simulink model "C_sim"  (R2024b)
settings: Solver=VariableStepAuto  StartTime=0.0  StopTime=ncs.simTime  FixedStep=Td  RelTol=1e-3
InitFcn:
  | set_param(gcs, 'SimulationCommand', 'update')
values from neighbouring files (symbols this model uses):
  ncs = NcsStructure(ncsPlant, 'simTime', simulationTime, 'controlParams', controlParams)    [main.m]
undefined symbols (not defined in the file or in its folder): sfunchk
libraries: cstblocks x1, truetime x1
settings Model: Creator=jakob_ludwiger  LastModifiedBy=proph37
settings SolverCC: AlgebraicLoopSolver=TrustRegion
settings DataIOCC: ReturnWorkspaceOutputs=off
settings DebuggingCC: UnconnectedInputMsg=warning  UnconnectedOutputMsg=warning  UnconnectedLineMsg=warning  ArithmeticOperatorsInVariantConditions=warning
settings ModelReferenceCC: EnableRefExpFcnMdlSchedulingChecks=on
settings SFSimCC: SimUseLocalCustomCode=off  CustomCodeUndefinedFunction=UseInterfaceOnly
settings RTWCC: RTWUseLocalCustomCode=off  GPUComputeCapability=3.5  DLArmComputeVersion=19.05
settings CodeAppCC: StateflowObjectComments=on

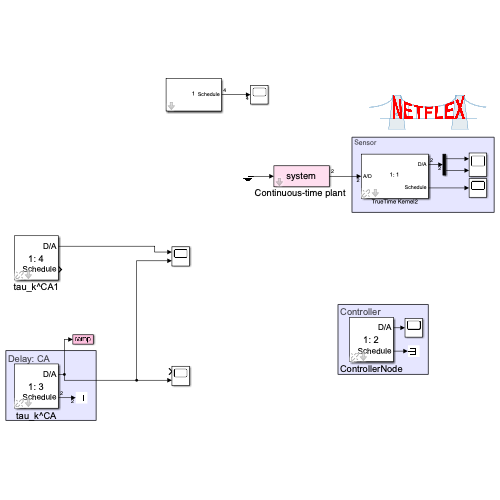
[thumbnail: Simulink's stored preview of the top-level diagram]
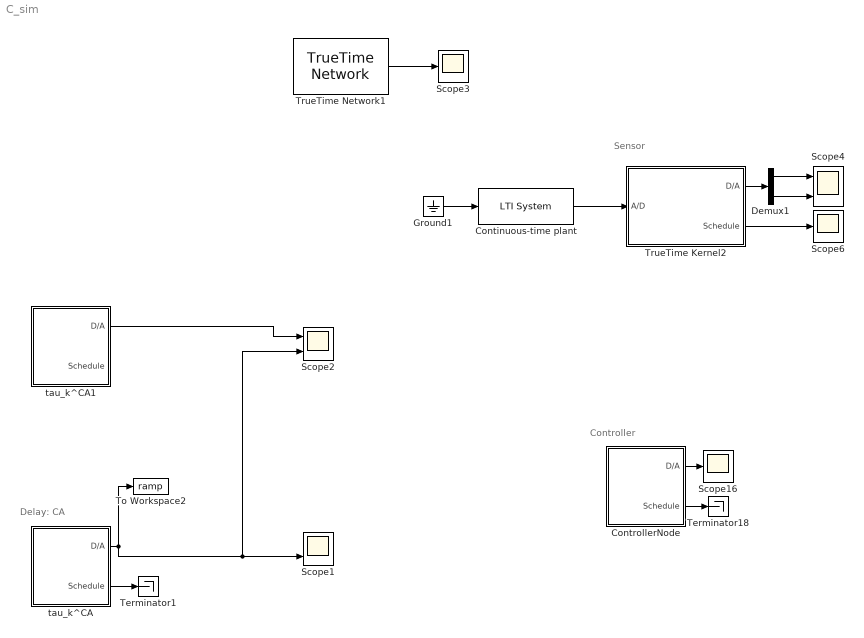
== system C_sim ==
  note: Controller
  note: Sensor
  note: Delay: CA
  "Continuous-time plant " : cstblocks/LTI System  sys=system  IC=initialState  PadeOrder=0
  ControllerNode : Subsystem  AncestorBlock=truetime/TrueTime Kernel  InitFcn=sfunchk(get_param(gcb,'sfun'));  mask{nodeObj=ncs.controllerNode, sfun=initFctWrapper, ntriggers=0, trigtype=falling, clockoffsetdrift=[0 0], schedoutput=on, battery=off, poweroutput=off, label=1: 2}
      mask prompts: nodeObj "Node Object"; sfun "Name of init function (MEX or MATLAB):"; ntriggers "Number of external triggers:"; trigtype "Trigger type:"; clockoffsetdrift "Local clock offset and drift:"; schedoutput "Show Schedule output port"; battery "Show Energy supply input port"; poweroutput "Show Power consumption output port"
      mask init:
      | set_param(gcb,'sfun', nodeObj.initFunctionWrapper)
      | %set_param(gcb,'args', [3 2])
      | args = nodeObj;
      | ninputsoutputs = [nodeObj.Nin nodeObj.Nout];
      | nwnodenbr = nodeObj.nodenumber;
      | ttkernel_callback(gcb,{sfun,args,ninputsoutputs,ntriggers,trigtype,nwnodenbr,clockoffsetdrift,schedoutput,battery,poweroutput})
      settings: ErrorFcn=ttkernel_error
      mask TypeOptions trigtype: rising | falling | either
      mask Display: disp(get_param(gcb,'label'))
  Demux1 : Demux  Outputs=2
  Ground1 : Ground
  Scope1 : Scope  NumInputPorts=2
  Scope16 : Scope
  Scope2 : Scope  NumInputPorts=2
  Scope3 : Scope
  Scope4 : Scope  NumInputPorts=2
  Scope6 : Scope
  Terminator1 : Terminator
  Terminator18 : Terminator
  To Workspace2 : ToWorkspace  VariableName=ramp  SaveFormat=Timeseries  SampleTime=1e-5
  TrueTime Kernel2 : Subsystem  AncestorBlock=truetime/TrueTime Kernel  InitFcn=sfunchk(get_param(gcb,'sfun'));  mask{nodeObj=ncs.sensorNode, sfun=initFctWrapper, ntriggers=0, trigtype=falling, clockoffsetdrift=[0 0], schedoutput=on, battery=off, poweroutput=off, label=1: 1}
      mask prompts: nodeObj "Node Object"; sfun "Name of init function (MEX or MATLAB):"; ntriggers "Number of external triggers:"; trigtype "Trigger type:"; clockoffsetdrift "Local clock offset and drift:"; schedoutput "Show Schedule output port"; battery "Show Energy supply input port"; poweroutput "Show Power consumption output port"
      mask init: same as C_sim/ControllerNode
      settings: ErrorFcn=ttkernel_error
      mask TypeOptions trigtype: rising | falling | either
      mask Display: disp(get_param(gcb,'label'))
  TrueTime Network1 : truetime/TrueTime Network  nwtype=CSMA/CD (Ethernet)  nwnbr=1  nnodes=ncs.getMaxNodeNumber  rate=1e8  minsize=200  lossprob=0  seed=0  bandwidths=[0.5 0.5]  slotsize=512  schedule=[1 1 2]  memsize=80000  buftype=Common buffer  overflow=Retransmit  dynSchedule=0  miniSlotSize=0  NIT=0  QSortMode=FIFO  sync=0  irtSchedule=0  nrtLength=0  nodeGraph=0  scheduleoutput=on
  tau_k^CA : Subsystem  AncestorBlock=truetime/TrueTime Kernel  InitFcn=sfunchk(get_param(gcb,'sfun'));  mask{nodeObj=ncs.tauCaNode, sfun=initFctWrapper, ntriggers=0, trigtype=falling, clockoffsetdrift=[0 0], schedoutput=on, battery=off, poweroutput=off, label=1: 3}
      mask prompts: nodeObj "Node Object"; sfun "Name of init function (MEX or MATLAB):"; ntriggers "Number of external triggers:"; trigtype "Trigger type:"; clockoffsetdrift "Local clock offset and drift:"; schedoutput "Show Schedule output port"; battery "Show Energy supply input port"; poweroutput "Show Power consumption output port"
      mask init: same as C_sim/ControllerNode
      settings: ErrorFcn=ttkernel_error
      mask TypeOptions trigtype: rising | falling | either
      mask Display: disp(get_param(gcb,'label'))
  tau_k^CA1 : Subsystem  AncestorBlock=truetime/TrueTime Kernel  InitFcn=sfunchk(get_param(gcb,'sfun'));  mask{nodeObj=ncs.test1, sfun=initFctWrapper, ntriggers=0, trigtype=falling, clockoffsetdrift=[0 0], schedoutput=on, battery=off, poweroutput=off, label=1: 4}
      mask prompts: nodeObj "Node Object"; sfun "Name of init function (MEX or MATLAB):"; ntriggers "Number of external triggers:"; trigtype "Trigger type:"; clockoffsetdrift "Local clock offset and drift:"; schedoutput "Show Schedule output port"; battery "Show Energy supply input port"; poweroutput "Show Power consumption output port"
      mask init: same as C_sim/ControllerNode
      settings: ErrorFcn=ttkernel_error
      mask TypeOptions trigtype: rising | falling | either
      mask Display: disp(get_param(gcb,'label'))
  wires:
  TrueTime Network1/1 -> Scope3/1
  TrueTime Kernel2/2(Schedule) -> Scope6/1
  Demux1/2 -> Scope4/2
  Ground1/1 -> "Continuous-time plant "/1
  ControllerNode/1(D/A) -> Scope16/1
  "Continuous-time plant "/1 -> TrueTime Kernel2/1(A/D)
  ControllerNode/2(Schedule) -> Terminator18/1
  TrueTime Kernel2/1(D/A) -> Demux1/1
  Demux1/1 -> Scope4/1
  tau_k^CA/1(D/A) -> To Workspace2/1, Scope2/2, Scope1/2
  tau_k^CA/2(Schedule) -> Terminator1/1
  tau_k^CA1/1(D/A) -> Scope2/1

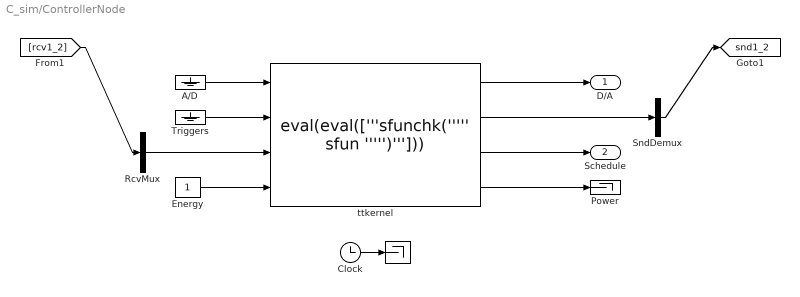
== system C_sim/ControllerNode ==
  " " : Terminator
  A/D : Ground
  Clock : Clock
  Energy : Constant
  Power : Terminator
  RcvMux : Mux  Inputs=1
  SndDemux : Demux  Outputs=1
      settings: DisplayOption=none
  Triggers : Ground
  ttkernel : S-Function  FunctionName=eval(eval(['''sfunchk(''''' sfun ''''')''']))  Parameters=sfun, args, ninputsoutputs, ntriggers, trigtype, nwnodenbr, clockoffsetdrift  SFunctionDeploymentMode=off  EnableBusSupport=off
  D/A : Outport
  Schedule : Outport  Port=2
  tag scope: snd1_2=global
  wires:
  Clock/1 -> " "/1
  RcvMux/1 -> ttkernel/3
  Triggers/1 -> ttkernel/2
  ttkernel/3 -> Schedule/1
  ttkernel/1 -> D/A/1
  ttkernel/2 -> SndDemux/1
  A/D/1 -> ttkernel/1
  Energy/1 -> ttkernel/4
  ttkernel/4 -> Power/1
  [rcv1_2] -> RcvMux/1
  SndDemux/1 -> [snd1_2]

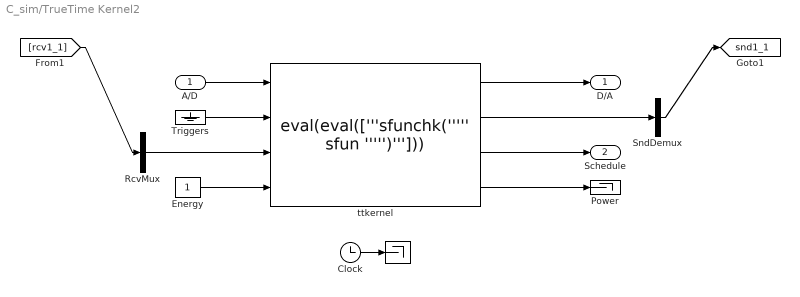
== system C_sim/TrueTime Kernel2 ==
  A/D : Inport
  " " : Terminator
  Clock : Clock
  Energy : Constant
  Power : Terminator
  RcvMux : Mux  Inputs=1
  SndDemux : Demux  Outputs=1
      settings: DisplayOption=none
  Triggers : Ground
  ttkernel : S-Function  FunctionName=eval(eval(['''sfunchk(''''' sfun ''''')''']))  Parameters=sfun, args, ninputsoutputs, ntriggers, trigtype, nwnodenbr, clockoffsetdrift  SFunctionDeploymentMode=off  EnableBusSupport=off
  D/A : Outport
  Schedule : Outport  Port=2
  tag scope: snd1_1=global
  wires:
  ttkernel/4 -> Power/1
  Energy/1 -> ttkernel/4
  A/D/1 -> ttkernel/1
  ttkernel/2 -> SndDemux/1
  ttkernel/1 -> D/A/1
  ttkernel/3 -> Schedule/1
  Triggers/1 -> ttkernel/2
  RcvMux/1 -> ttkernel/3
  Clock/1 -> " "/1
  [rcv1_1] -> RcvMux/1
  SndDemux/1 -> [snd1_1]

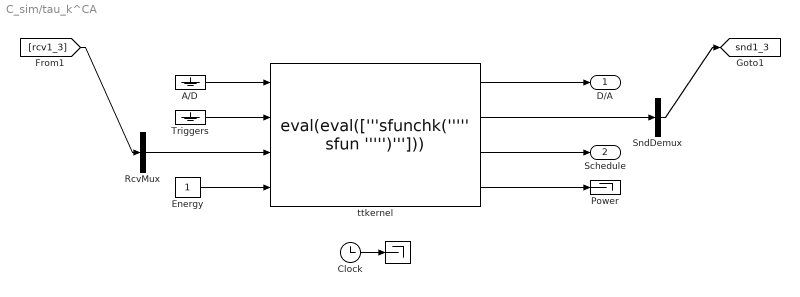
== system C_sim/tau_k^CA ==
  " " : Terminator
  A/D : Ground
  Clock : Clock
  Energy : Constant
  Power : Terminator
  RcvMux : Mux  Inputs=1
  SndDemux : Demux  Outputs=1
      settings: DisplayOption=none
  Triggers : Ground
  ttkernel : S-Function  FunctionName=eval(eval(['''sfunchk(''''' sfun ''''')''']))  Parameters=sfun, args, ninputsoutputs, ntriggers, trigtype, nwnodenbr, clockoffsetdrift  SFunctionDeploymentMode=off  EnableBusSupport=off
  D/A : Outport
  Schedule : Outport  Port=2
  tag scope: snd1_3=global
  wires:
  ttkernel/4 -> Power/1
  Energy/1 -> ttkernel/4
  A/D/1 -> ttkernel/1
  ttkernel/2 -> SndDemux/1
  ttkernel/1 -> D/A/1
  ttkernel/3 -> Schedule/1
  Triggers/1 -> ttkernel/2
  RcvMux/1 -> ttkernel/3
  Clock/1 -> " "/1
  [rcv1_3] -> RcvMux/1
  SndDemux/1 -> [snd1_3]

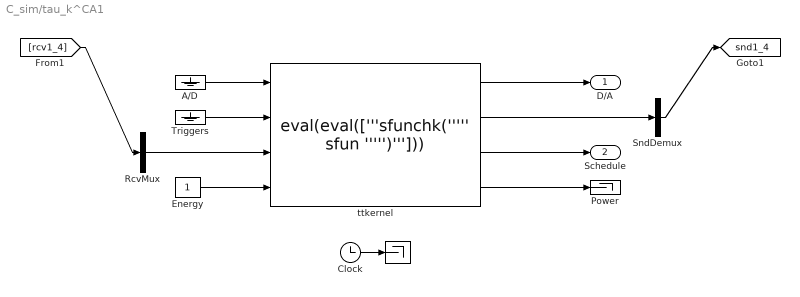
== system C_sim/tau_k^CA1 ==
  " " : Terminator
  A/D : Ground
  Clock : Clock
  Energy : Constant
  Power : Terminator
  RcvMux : Mux  Inputs=1
  SndDemux : Demux  Outputs=1
      settings: DisplayOption=none
  Triggers : Ground
  ttkernel : S-Function  FunctionName=eval(eval(['''sfunchk(''''' sfun ''''')''']))  Parameters=sfun, args, ninputsoutputs, ntriggers, trigtype, nwnodenbr, clockoffsetdrift  SFunctionDeploymentMode=off  EnableBusSupport=off
  D/A : Outport
  Schedule : Outport  Port=2
  tag scope: snd1_4=global
  wires:
  ttkernel/4 -> Power/1
  Energy/1 -> ttkernel/4
  A/D/1 -> ttkernel/1
  ttkernel/2 -> SndDemux/1
  ttkernel/1 -> D/A/1
  ttkernel/3 -> Schedule/1
  Triggers/1 -> ttkernel/2
  RcvMux/1 -> ttkernel/3
  Clock/1 -> " "/1
  [rcv1_4] -> RcvMux/1
  SndDemux/1 -> [snd1_4]
